simulink model "Fadhlan_Firasyan_Data_Driven_Modelling_30Sep2024"  (R2023a)
settings: Solver=VariableStepAuto  StartTime=0.0  StopTime=10.0  RelTol=1e-3
undefined symbols (not defined in the file): Ts1, Ts2
settings Model: Creator=HP  LastModifiedBy=HP

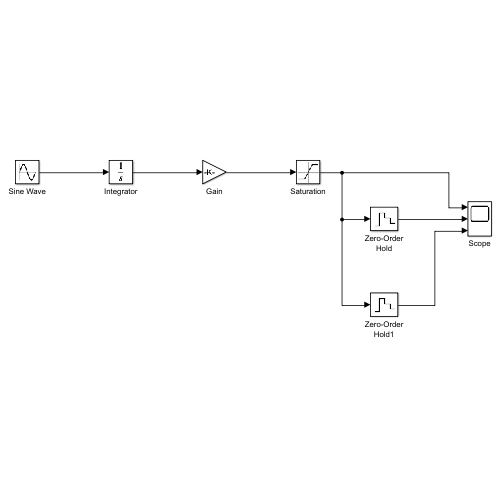
[thumbnail: Simulink's stored preview of the top-level diagram]
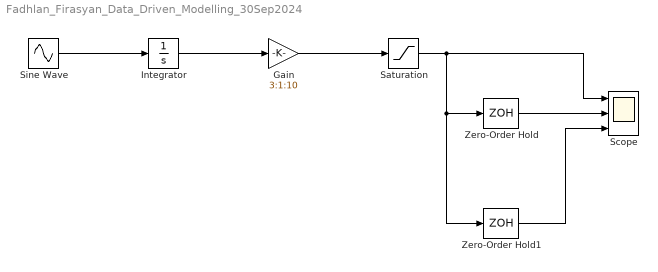
== system Fadhlan_Firasyan_Data_Driven_Modelling_30Sep2024 ==
  Gain : Gain  Gain=3:1:10
  Integrator : Integrator
  Saturation : Saturate  UpperLimit=rand(8,1)*10  LowerLimit=rand(8,1)*-10
  Scope : Scope  NumInputPorts=3
  Sine Wave : Sin  SampleTime=0
  Zero-Order Hold : ZeroOrderHold  SampleTime=Ts1
  Zero-Order Hold1 : ZeroOrderHold  SampleTime=Ts2
  wires:
  Sine Wave/1 -> Integrator/1
  Integrator/1 -> Gain/1
  Gain/1 -> Saturation/1
  Saturation/1 -> Zero-Order Hold/1, Zero-Order Hold1/1, Scope/1
  Zero-Order Hold/1 -> Scope/2
  Zero-Order Hold1/1 -> Scope/3
